simulink model "solar_powered_battery_with_Boost_MPPT"  (R2021a)
settings: Solver=VariableStepAuto  StartTime=0.0  StopTime=2  RelTol=1e-3
libraries: spsSeriesRLCBranchLib x4, spsDiodeLib x1, spsIGBTDiodeLib x1, spsPWMGeneratorDCDCLib x1, spsControlledCurrentSourceLib x1, spsVoltageMeasurementLib x1, spspowerguiLib x1
settings Model: Creator=76568  LastModifiedBy=76568

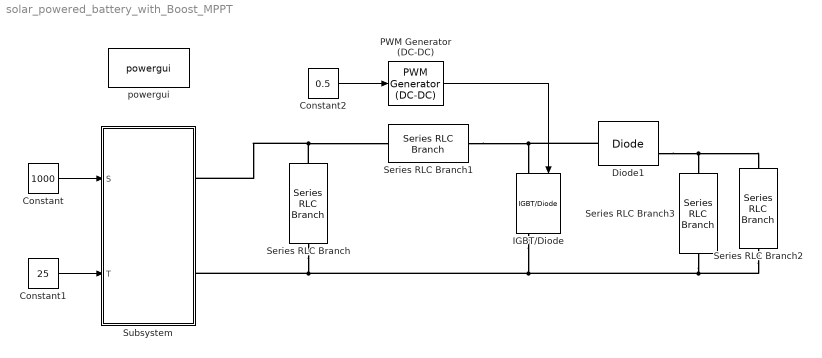
== system solar_powered_battery_with_Boost_MPPT ==
  Constant : Constant  Value=1000
  Constant1 : Constant  Value=25
  Constant2 : Constant  Value=0.5
  Diode1 : spsDiodeLib/Diode  Ron=0.001  Lon=0  Vf=0.8  IC=0  UseSnubber=0  Rs=500  Cs=250e-9  Measurements=on
  IGBT/Diode : spsIGBTDiodeLib/IGBT//Diode  Ron=1e-3  Rs=1e5  Cs=inf  Measurements=on
  PWM Generator (DC-DC) : spsPWMGeneratorDCDCLib/PWM Generator (DC-DC)  Fsw=12e3  Ts=0
  Series RLC Branch : spsSeriesRLCBranchLib/Series RLC Branch  LConnTagsString=__new0  RConnTagsString=__new0  BranchType=C  Resistance=1  Inductance=1e-3  SetiL0=off  InitialCurrent=0  Capacitance=1e-3  Setx0=off  InitialVoltage=0  Measurements=None
  Series RLC Branch1 : spsSeriesRLCBranchLib/Series RLC Branch  LConnTagsString=__new0  RConnTagsString=__new0  BranchType=L  Resistance=1  Inductance=1e-3  SetiL0=off  InitialCurrent=0  Capacitance=1e-3  Setx0=off  InitialVoltage=0  Measurements=None
  Series RLC Branch2 : spsSeriesRLCBranchLib/Series RLC Branch  LConnTagsString=__new0  RConnTagsString=__new0  BranchType=R  Resistance=2  Inductance=1e-3  SetiL0=off  InitialCurrent=0  Capacitance=1e-3  Setx0=off  InitialVoltage=0  Measurements=None
  Series RLC Branch3 : spsSeriesRLCBranchLib/Series RLC Branch  LConnTagsString=__new0  RConnTagsString=__new0  BranchType=C  Resistance=1  Inductance=1e-3  SetiL0=off  InitialCurrent=0  Capacitance=1e-3  Setx0=off  InitialVoltage=0  Measurements=None
  Subsystem : Subsystem  mask{Uoc=14.5, Um=11.9, Isc=5.5, Im=5.3}
  powergui : spspowerguiLib/powergui  Priority=1  SimulationMode=Continuous  SampleTime=1/12e3/50  frequency=60  Iterations=50  frequencyindice=0  Pbase=100e6  ErrMax=1e-4  UnitsV=kV  UnitsW=MW  buscounter=0  FunctionMessages=off  echomessages=off  EnableUseOfTLC=off  CurrentSourceSwitches=off  DisableSnubberDevices=off  DisableRonSwitches=off  DisableVfSwitches=off  DisplayEquations=off  AutomaticDiscreteSolvers=off  SolverType=Tustin/Backward Euler (TBE)  Interpol=off  ExternalGateDelay=off  methode=off  Ts=100  x0status=blocks  SPID=on  SwTol=0  HookPort=off  NonlinearTolerance=1e-4  nMaxIteration=100  ContinueOnMaxIteration=off  RestoreLinks=warning  ResistiveCurrentMeasurement=off  Frange=[0:2:500]  Ylog=off  Xlog=on  ShowGrid=off  save=off  variable=ZData  structure=0  ZoomFFT=off  StartTime=0.0  cycles=1  DisplayStyle=1  fundamental=60  FreqAxis=off  MaxFrequency=1000  frequencyindicesteady=1  RmsSteady=1  display=off
  wires:
  PWM Generator (DC-DC)/1 -> IGBT/Diode/1
  Constant1/1 -> Subsystem/2(T)
  Constant/1 -> Subsystem/1(S)
  Constant2/1 -> PWM Generator (DC-DC)/1
  connections:
  Series RLC Branch1/RConn1 -- Diode1/LConn1 -- IGBT/Diode/LConn1
  Series RLC Branch3/RConn1 -- Series RLC Branch2/RConn1 -- IGBT/Diode/RConn1 -- Subsystem/RConn2 -- Series RLC Branch/RConn1
  Series RLC Branch/LConn1 -- Subsystem/RConn1 -- Series RLC Branch1/LConn1
  Diode1/RConn1 -- Series RLC Branch2/LConn1 -- Series RLC Branch3/LConn1

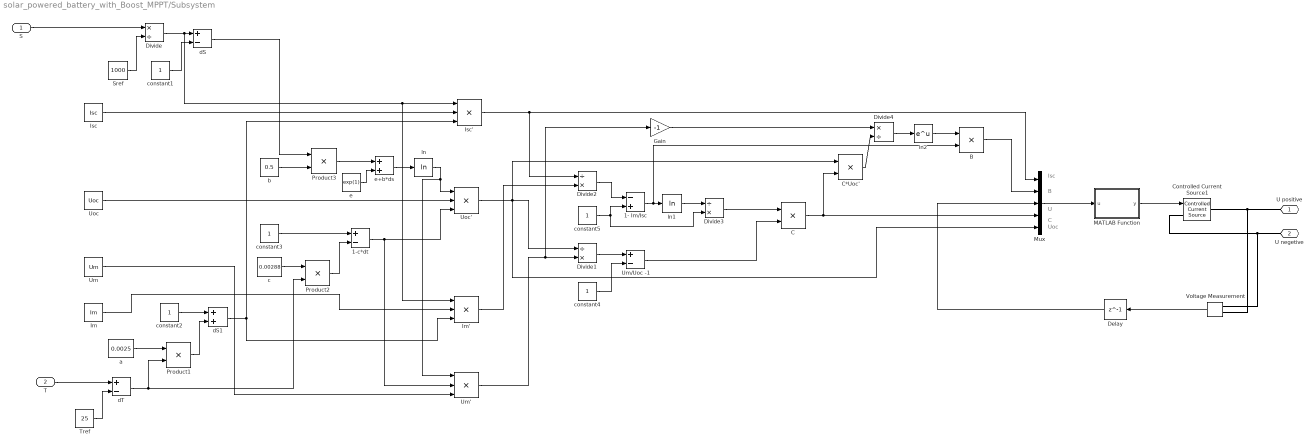
== system solar_powered_battery_with_Boost_MPPT/Subsystem ==
  note: Isc
  note: B
  note: U
  note: C
  note: Uoc
  S : Inport
  T : Inport  Port=2
  1- Im/Isc : Sum  Inputs=-+
  1-c*dt : Sum  Inputs=+-
  B : Product
  C : Product
  C*Uoc' : Product
  Controlled Current Source1 : spsControlledCurrentSourceLib/Controlled Current Source  Initialize=on  Source_Type=DC  Amplitude=0  Phase=0  Frequency=0  Measurements=None
  Delay : Delay  DelayLength=1  InitialCondition=0  SampleTime=0.0001
  Divide : Product  Inputs=*/
  Divide1 : Product  Inputs=/*
  Divide2 : Product  Inputs=/*
  Divide3 : Product  Inputs=/*
  Divide4 : Product  Inputs=*/
  Gain : Gain  Gain=-1
  Im : Constant  Value=Im
  Im' : Product  Inputs=3
  Isc : Constant  Value=Isc
  Isc' : Product  Inputs=3
  MATLAB Function : MATLAB Function  TreatAsAtomicUnit=on
  Mux : Mux  Inputs=5
  Product1 : Product
  Product2 : Product
  Product3 : Product
  Sref : Constant  Value=1000
  Tref : Constant  Value=25
  Um : Constant  Value=Um
  Um' : Product  Inputs=3
  Um/Uoc -1 : Sum  Inputs=+-
  Uoc : Constant  Value=Uoc
  Uoc' : Product  Inputs=3
  Voltage Measurement : spsVoltageMeasurementLib/Voltage Measurement  PhasorSimulation=off  OutputType=Complex  PSBequivalent=0
  a : Constant  Value=0.0025
  b : Constant  Value=0.5
  c : Constant  Value=0.00288
  constant{1..5} (5 alike) : Constant
  dS : Sum  Inputs=+-
  dS1 : Sum
  dT : Sum  Inputs=+-
  e : Constant  Value=exp(1)
  e+b*ds : Sum
  ln : Math  Operator=log  SaturateOnIntegerOverflow=on
  ln1 : Math  Operator=log  SaturateOnIntegerOverflow=on
  ln2 : Math  SaturateOnIntegerOverflow=on
  U positive : PMIOPort  Side=Right
  U negetive : PMIOPort  Port=2  Side=Right
  wires:
  Mux/1 -> MATLAB Function/1(u)
  T/1 -> dT/1
  Tref/1 -> dT/2
  S/1 -> Divide/1
  Sref/1 -> Divide/2
  Divide/1 -> Isc'/1, Im'/1, dS/1
  constant1/1 -> dS/2
  a/1 -> Product1/1
  dT/1 -> Product2/2, Product1/2
  constant2/1 -> dS1/1
  Product1/1 -> dS1/2
  dS1/1 -> Im'/3, Isc'/3
  Isc/1 -> Isc'/2
  Uoc/1 -> Uoc'/2
  constant3/1 -> 1-c*dt/1
  Product2/1 -> 1-c*dt/2
  c/1 -> Product2/1
  1-c*dt/1 -> Um'/2, Uoc'/3
  b/1 -> Product3/2
  dS/1 -> Product3/1
  e/1 -> e+b*ds/2
  Product3/1 -> e+b*ds/1
  e+b*ds/1 -> ln/1
  ln/1 -> Um'/1, Uoc'/1
  Im/1 -> Im'/2
  Um/1 -> Um'/3
  Um'/1 -> Gain/1, Divide1/2
  Divide1/1 -> Um/Uoc -1/1
  constant4/1 -> Um/Uoc -1/2
  Im'/1 -> Divide2/2
  Isc'/1 -> Mux/1, Divide2/1
  Divide2/1 -> 1- Im/Isc/1
  constant5/1 -> Divide3/2, 1- Im/Isc/2
  1- Im/Isc/1 -> B/2, ln1/1
  ln1/1 -> Divide3/1
  Um/Uoc -1/1 -> C/2
  Divide3/1 -> C/1
  C/1 -> C*Uoc'/2, Mux/4
  Gain/1 -> Divide4/1
  C*Uoc'/1 -> Divide4/2
  Divide4/1 -> ln2/1
  ln2/1 -> B/1
  B/1 -> Mux/2
  Voltage Measurement/1 -> Delay/1
  Delay/1 -> Mux/3
  Uoc'/1 -> Mux/5, Divide1/1, C*Uoc'/1
  MATLAB Function/1(y) -> Controlled Current Source1/1
  connections:
  Voltage Measurement/LConn2 -- U negetive/RConn1 -- Controlled Current Source1/LConn1
  Voltage Measurement/LConn1 -- U positive/RConn1 -- Controlled Current Source1/RConn1

== matlab function solar_powered_battery_with_Boost_MPPT/Subsystem/MATLAB Function ==
  data: u input; y output
function y = fcn(u)
y=u(1)*(1-u(2)*(exp(u(3)/u(4)/u(5))-1));
